simulink model "LV5_PI_regulator_ZN2"  (R2018a)
settings: Solver=ode45  StartTime=0.0  StopTime=t_sim  RelTol=1e-5
undefined symbols (not defined in the file): A1, A2, g, h10, h20, Kh, Ki, Km, Kpi, Kv, qu0, t_step, Tv, u0
settings Model: Creator=Mislav  LastModifiedBy=Mislav
settings SFSimCC: SimUseLocalCustomCode=on
settings RTWCC: RTWUseLocalCustomCode=on

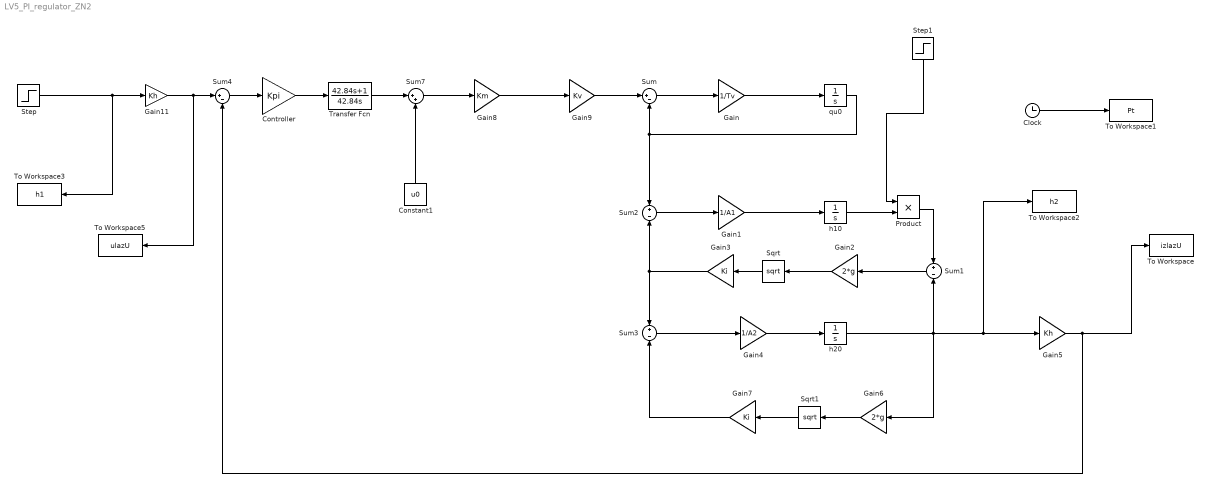
== system LV5_PI_regulator_ZN2 ==
  Clock : Clock
  Constant1 : Constant  Value=u0
  Controller : Gain  Gain=Kpi
  Gain : Gain  Gain=1/Tv
  Gain1 : Gain  Gain=1/A1
  Gain11 : Gain  Gain=Kh
  Gain2 : Gain  Gain=2*g
  Gain3 : Gain  Gain=Ki
  Gain4 : Gain  Gain=1/A2
  Gain5 : Gain  Gain=Kh
  Gain6 : Gain  Gain=2*g
  Gain7 : Gain  Gain=Ki
  Gain8 : Gain  Gain=Km
  Gain9 : Gain  Gain=Kv
  Product : Product
  Sqrt : Sqrt  SaturateOnIntegerOverflow=on
  Sqrt1 : Sqrt  SaturateOnIntegerOverflow=on
  Step : Step  Time=t_step  Before=h20  After=h20*1.1  SampleTime=0
  Step1 : Step  Time=900  Before=1  After=1.02  SampleTime=0
  Sum : Sum  Inputs=|+-
  Sum1 : Sum  Inputs=+-
  Sum2 : Sum  Inputs=+|-
  Sum3 : Sum  Inputs=+|-
  Sum4 : Sum  Inputs=|+-
  Sum7 : Sum  Inputs=|++
  To Workspace : ToWorkspace  VariableName=izlazU  SampleTime=-1
      settings: Save2DSignal=2-D array (concatenate along first dimension)
  To Workspace1 : ToWorkspace  VariableName=Pt  SampleTime=-1
      settings: Save2DSignal=2-D array (concatenate along first dimension)
  To Workspace2 : ToWorkspace  VariableName=h2  SampleTime=-1
      settings: Save2DSignal=2-D array (concatenate along first dimension)
  To Workspace3 : ToWorkspace  VariableName=h1  SampleTime=-1
      settings: Save2DSignal=2-D array (concatenate along first dimension)
  To Workspace5 : ToWorkspace  VariableName=ulazU  SampleTime=-1
      settings: Save2DSignal=2-D array (concatenate along first dimension)
  Transfer Fcn : TransferFcn  Numerator=[42.84 1]  Denominator=[42.84 0]
  "h10 " : Integrator  InitialCondition=h10
  "h20 " : Integrator  InitialCondition=h20
  "qu0 " : Integrator  InitialCondition=qu0
  wires:
  Gain/1 -> "qu0 "/1
  "qu0 "/1 -> Sum/2, Sum2/1
  Transfer Fcn/1 -> Sum7/1
  Gain4/1 -> "h20 "/1
  "h20 "/1 -> Gain6/1, To Workspace2/1, Gain5/1, Sum1/2
  Gain2/1 -> Sqrt/1
  Gain6/1 -> Sqrt1/1
  Gain7/1 -> Sum3/2
  Sum4/1 -> Controller/1
  Sqrt1/1 -> Gain7/1
  Sum3/1 -> Gain4/1
  Constant1/1 -> Sum7/2
  Sum2/1 -> Gain1/1
  Gain1/1 -> "h10 "/1
  Clock/1 -> To Workspace1/1
  Gain11/1 -> Sum4/1, To Workspace5/1
  Gain3/1 -> Sum2/2, Sum3/1
  Step/1 -> Gain11/1, To Workspace3/1
  Gain8/1 -> Gain9/1
  Sum7/1 -> Gain8/1
  Sqrt/1 -> Gain3/1
  Controller/1 -> Transfer Fcn/1
  Sum/1 -> Gain/1
  Gain9/1 -> Sum/1
  Gain5/1 -> To Workspace/1, Sum4/2
  Sum1/1 -> Gain2/1
  Step1/1 -> Product/1
  "h10 "/1 -> Product/2
  Product/1 -> Sum1/1
